simulink model "missile"  (R2019b)
settings: Solver=ode4  StartTime=0.0  StopTime=5  FixedStep=1e-4  MaxStep=0.01  RelTol=1e-4  EnableMultiTasking=on
values from neighbouring files (symbols this model uses):
  K = ss(zeros(2),eye(2),[2,2.5;1.5,2]/100,[2,2.5;1.5,2])    [Demo_010.m]    (also in Demo_013.m = null(Wi-C'/H*C); Demo_015.m = ss(aK,bK,cK,dK)*diag(diag(Jnom)))
  olic = sysic    [Demo_003.m]    (also in Demo_009.m; Demo_012.m = Usamp(:,:,i,1); Demo_014.m; Demo_015.m)
undefined symbols (not defined in the file or in its folder): sigbuilder_block
settings Model: Creator=Joost Veenman  LastModifiedBy=joost.veenman
settings DataIOCC: LimitDataPoints=on  SaveFormat=Array  SignalLoggingSaveFormat=ModelDataLogs  ReturnWorkspaceOutputs=off
settings OptimizationCC: ExpressionDepthLimit=2147483647  InitFltsAndDblsToZero=on  LifeSpan=inf
settings DebuggingCC: UnderspecifiedInitializationDetection=Classic  MergeDetectMultiDrivingBlocksExec=none  SolverPrmCheckMsg=warning  FcnCallInpInsideContextMsg=warning  StateNameClashWarn=warning  SFUnexpectedBacktrackingDiag=warning  SFNoUnconditionalDefaultTransitionDiag=warning  SFExecutionAtInitializationDiag=none  ArithmeticOperatorsInVariantConditions=warning
settings HardwareCC: ProdBitPerPointer=32  ProdBitPerSizeT=32  ProdBitPerPtrDiffT=32  ProdLargestAtomicFloat=None  ProdIntDivRoundTo=Undefined  ProdEndianess=Unspecified  ProdWordSize=32  ProdHWDeviceType=32-bit Generic
settings ModelReferenceCC: PropagateSignalLabelsOutOfModel=off
settings SFSimCC: SimUseLocalCustomCode=off  SimParseCustomCode=off  CustomCodeUndefinedFunction=UseInterfaceOnly
settings RTWCC: RTWUseLocalCustomCode=off
settings CodeAppCC: StateflowObjectComments=on
settings GRTTargetCC: TargetLangStandard=C89/C90 (ANSI)  GeneratePreprocessorConditionals=Disable all  CombineOutputUpdateFcns=off  GRTInterface=on
settings ConfigComp: CovMetricSettings=dw  CovHtmlReporting=on  CovSaveCumulativeToWorkspaceVar=on  CovSaveSingleToWorkspaceVar=on  CovExternalEMLEnable=off

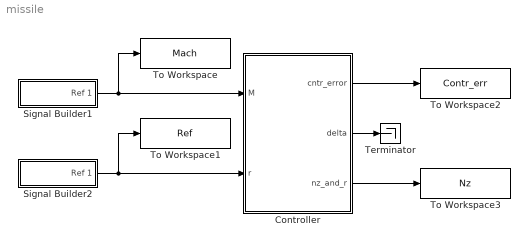
== system missile ==
  Controller : Subsystem
  Signal Builder1 : Subsystem  Tag=STV Subsys  LoadFcn=sigbuilder_block('load');  StartFcn=sigbuilder_block('start');  StopFcn=sigbuilder_block('stop');  ClipboardFcn=sigbuilder_block('clipboard');  mask(Sigbuilder block){tuvar=[0:10]}
      mask help: Sigbuilder GUI
      mask init:
      | if ~strcmp(get_param(bdroot(gcbh),'SimulationStatus'),'stopped') tuvar = sigbuilder_block('maskInit'); end
      settings: CopyFcn=sigbuilder_block('copy');  DeleteFcn=sigbuilder_block('delete');  ModelCloseFcn=sigbuilder_block('modelClose');  PreSaveFcn=sigbuilder_block('preSave');  PauseFcn=sigbuilder_block('pause')  ContinueFcn=sigbuilder_block('continue')  NameChangeFcn=sigbuilder_block('namechange');  OpenFcn=sigbuilder_block('open',[105.75 48 550.5 362.25 ]);  CloseFcn=sigbuilder_block('close');
      mask Display: plot(0, 0, 100, 100,[2, 2, 32, 32, 2], [68, 8, 8, 68, 68],[32, 2], [38, 38], [32, 19, 2],[53, 60, 44], [32, 17, 17, 2],[16, 16, 31, 31]);txt = getActiveGroup(gcbh);text(2, 100, txt,'verticalAlignment', 'top');
  Signal Builder2 : Subsystem  Tag=STV Subsys  LoadFcn=sigbuilder_block('load');  StartFcn=sigbuilder_block('start');  StopFcn=sigbuilder_block('stop');  ClipboardFcn=sigbuilder_block('clipboard');  mask(Sigbuilder block){tuvar=[0:10]}
      mask help: Sigbuilder GUI
      mask init:
      | if ~strcmp(get_param(bdroot(gcbh),'SimulationStatus'),'stopped') tuvar = sigbuilder_block('maskInit'); end
      settings: CopyFcn=sigbuilder_block('copy');  DeleteFcn=sigbuilder_block('delete');  ModelCloseFcn=sigbuilder_block('modelClose');  PreSaveFcn=sigbuilder_block('preSave');  PauseFcn=sigbuilder_block('pause')  ContinueFcn=sigbuilder_block('continue')  NameChangeFcn=sigbuilder_block('namechange');  OpenFcn=sigbuilder_block('open',[211.5 84 550.5 362.25 ]);  CloseFcn=sigbuilder_block('close');
      mask Display: plot(0, 0, 100, 100,[2, 2, 32, 32, 2], [68, 8, 8, 68, 68],[32, 2], [38, 38], [32, 19, 2],[53, 60, 44], [32, 17, 17, 2],[16, 16, 31, 31]);txt = getActiveGroup(gcbh);text(2, 100, txt,'verticalAlignment', 'top');
  Terminator : Terminator
  To Workspace : ToWorkspace  VariableName=Mach  SaveFormat=Timeseries  SampleTime=-1
  To Workspace1 : ToWorkspace  VariableName=Ref  SaveFormat=Timeseries  SampleTime=-1
  To Workspace2 : ToWorkspace  VariableName=Contr_err  SaveFormat=Timeseries  SampleTime=-1
  To Workspace3 : ToWorkspace  VariableName=Nz  SaveFormat=Timeseries  SampleTime=-1
  wires:
  Signal Builder2/1(Ref 1) -> Controller/2(r), To Workspace1/1
  Controller/1(cntr_error) -> To Workspace2/1
  Signal Builder1/1(Ref 1) -> Controller/1(M), To Workspace/1
  Controller/3(nz_and_r) -> To Workspace3/1
  Controller/2(delta) -> Terminator/1

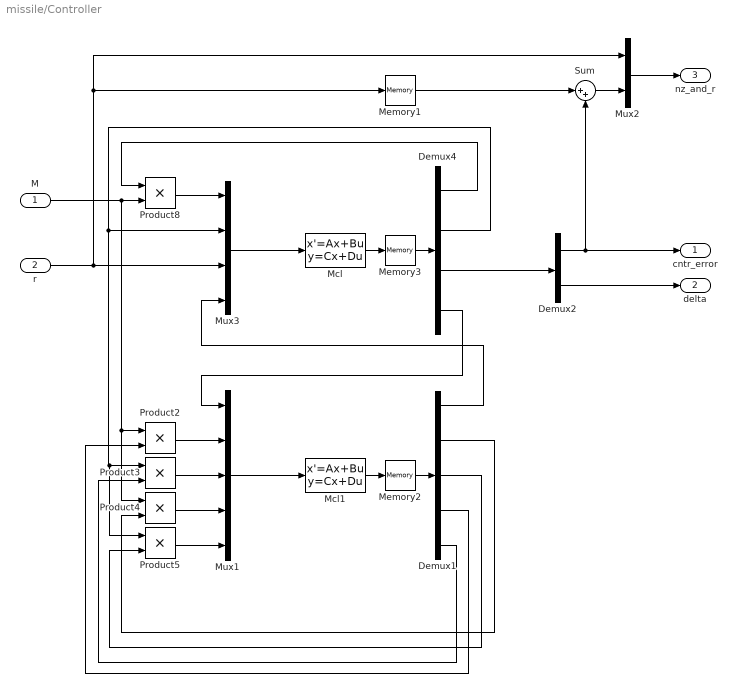
== system missile/Controller ==
  M : Inport
  r : Inport  Port=2
  Demux1 : Demux  Outputs=[1,5,2,5,2]
  Demux2 : Demux  Outputs=[1,1]
  Demux4 : Demux  Outputs=[5,2,2,2]
  Mcl : StateSpace  A=olic.a  B=olic.b  C=olic.c  D=olic.d  InitialCondition=0
  Mcl1 : StateSpace  A=K.a  B=K.b  C=K.c  D=K.d  InitialCondition=0
  Memory1 : Memory
  Memory2 : Memory
  Memory3 : Memory
  Mux1 : Mux  Inputs=[2,5,2,5,2]
  Mux2 : Mux  Inputs=[1,1]
  Mux3 : Mux  Inputs=[5,2,1,1]
  Product{2..5,8} (5 alike) : Product  RndMeth=Zero
  Sum : Sum  Inputs=|++
  cntr_error : Outport
  delta : Outport  Port=2
  nz_and_r : Outport  Port=3
  wires:
  Mux3/1 -> Mcl/1
  Product8/1 -> Mux3/1
  r/1 -> Mux2/1, Memory1/1, Mux3/3
  Mux1/1 -> Mcl1/1
  M/1 -> Product4/1, Product2/1, Product8/2
  Demux4/1 -> Product8/1
  Product2/1 -> Mux1/2
  Product3/1 -> Mux1/3
  Product4/1 -> Mux1/4
  Product5/1 -> Mux1/5
  Demux1/2 -> Product4/2
  Demux1/3 -> Product5/2
  Demux1/4 -> Product2/2
  Demux1/5 -> Product3/2
  Demux4/3 -> Demux2/1
  Demux2/1 -> cntr_error/1, Sum/2
  Demux2/2 -> delta/1
  Sum/1 -> Mux2/2
  Mux2/1 -> nz_and_r/1
  Mcl/1 -> Memory3/1
  Mcl1/1 -> Memory2/1
  Demux4/2 -> Product5/1, Product3/1, Mux3/2
  Demux1/1 -> Mux3/4
  Demux4/4 -> Mux1/1
  Memory2/1 -> Demux1/1
  Memory3/1 -> Demux4/1
  Memory1/1 -> Sum/1

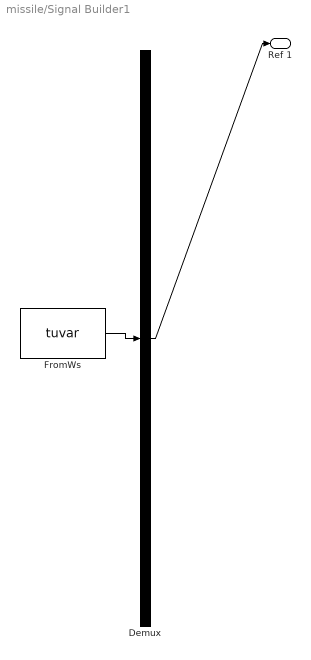
== system missile/Signal Builder1 ==
  Demux : Demux  Tag=STV Demux  Outputs=1
  FromWs : FromWorkspace  Tag=STV FromWs  VariableName=tuvar  SampleTime=0
      SigBuilderData=|
      | common.afterFinalStr = 'Extrapolate'
      | common.sampleTime = 0
      | dataSet.timeRange = [0 5]
      | dataSet.name = 'Group 1'
      | sbobj.Groups.Name = 'Group 1'
      | sbobj.Groups.Signals.Name = 'Ref 1'
      | sbobj.Groups.Signals.XData = [0 1 3 4 5]
      | sbobj.Groups.Signals.YData = [0.5 1 1 -1 -1]
      | sbobj.Groups.TimeRange = [0 5]
  Ref 1 : Outport  Tag=STV Outport
  wires:
  FromWs/1 -> Demux/1
  Demux/1 -> Ref 1/1

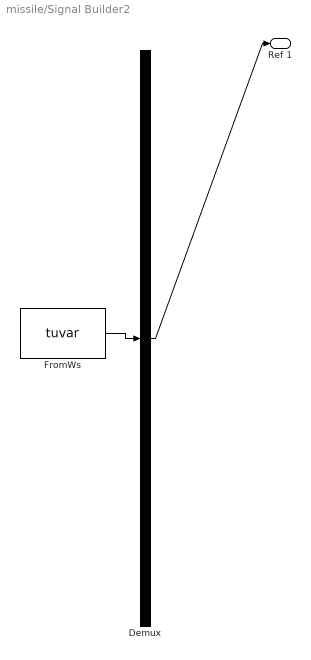
== system missile/Signal Builder2 ==
  Demux : Demux  Tag=STV Demux  Outputs=1
  FromWs : FromWorkspace  Tag=STV FromWs  VariableName=tuvar  SampleTime=0
      SigBuilderData=|
      | common.afterFinalStr = 'Extrapolate'
      | common.sampleTime = 0
      | dataSet.timeRange = [0 5]
      | dataSet.name = 'Group 1'
      | sbobj.Groups.Name = 'Group 1'
      | sbobj.Groups.Signals.Name = 'Ref 1'
      | sbobj.Groups.Signals.XData = [0 1 1 2 2 3 3 5]
      | sbobj.Groups.Signals.YData = [30 30 -15 -15 -10 -10 5 5]
      | sbobj.Groups.TimeRange = [0 5]
  Ref 1 : Outport  Tag=STV Outport
  wires:
  FromWs/1 -> Demux/1
  Demux/1 -> Ref 1/1
